simulink model "Triangle_Waveform"  (Simulink 7.8)
settings: Solver=ode45  StartTime=0.0  StopTime=10.0  FixedStep=0.0001  MaxStep=0.001  RelTol=1e-3
settings Model: Creator=VSH  LastModifiedBy=VSH

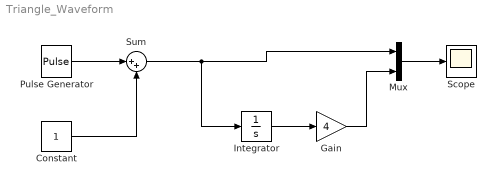
== system Triangle_Waveform ==
  Constant : Constant
  Gain : Gain  Gain=4
  Integrator : Integrator
  Mux : Mux  Inputs=2
  Pulse Generator : DiscretePulseGenerator  PulseType=Time based  Amplitude=-2  Period=1  PulseWidth=50  PhaseDelay=0.25
  Scope : Scope
      settings: MaxDataPoints=500000
  Sum : Sum  Inputs=|++
  wires:
  Mux/1 -> Scope/1
  Pulse Generator/1 -> Sum/1
  Constant/1 -> Sum/2
  Sum/1 -> Mux/1, Integrator/1
  Integrator/1 -> Gain/1
  Gain/1 -> Mux/2
